simulink model "Comparacao_continuo_discreto"  (R2023b)
settings: Solver=FixedStepAuto  StartTime=0.0  StopTime=3  FixedStep=T  RelTol=1e-3
model workspace (MAT data in the model file):
  B = 0.0928996133407
  Cmn = 479.991198073
  I = 3000
  Ian = 260.13143483
  J = 0.56
  Kf = 1.91586963478
  La = 0.0014
  N = 3000
  Pele = 104052.573932
  Pmec = 95000
  Ra = 0.08
  T = 0.00175
  Te = 0.0175
  Tm = 6.02801217209
  Vn = 400
  Wn = 197.920296
libraries: simulink x1
settings Model: Creator=lpds  LastModifiedBy=USER

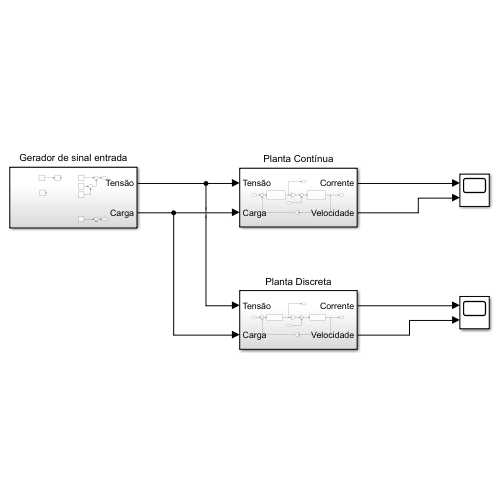
[thumbnail: Simulink's stored preview of the top-level diagram]
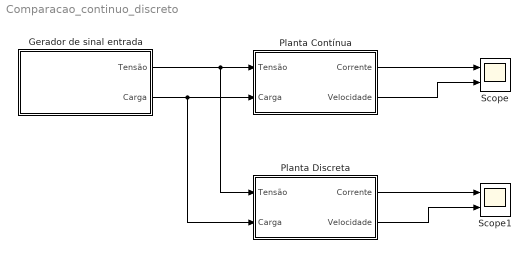
== system Comparacao_continuo_discreto ==
  Gerador de sinal entrada : Subsystem
  Planta Contínua : Subsystem
  Planta Discreta : Subsystem
  Scope : Scope  NumInputPorts=2
  Scope1 : Scope  NumInputPorts=2
  wires:
  Gerador de sinal entrada/1(Tensão) -> Planta Discreta/1(Tensão), Planta Contínua/1(Tensão)
  Gerador de sinal entrada/2(Carga) -> Planta Discreta/2(Carga), Planta Contínua/2(Carga)
  Planta Contínua/1(Corrente) -> Scope/1
  Planta Contínua/2(Velocidade) -> Scope/2
  Planta Discreta/1(Corrente) -> Scope1/1
  Planta Discreta/2(Velocidade) -> Scope1/2

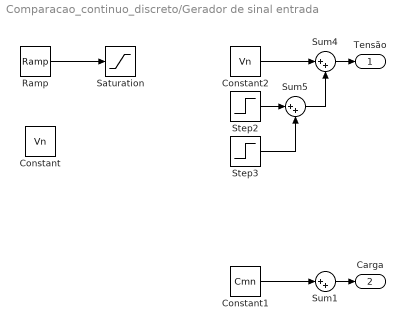
== system Comparacao_continuo_discreto/Gerador de sinal entrada ==
  Constant : Constant  Value=Vn
  Constant1 : Constant  Value=Cmn
  Constant2 : Constant  Value=Vn
  Ramp : simulink/Sources/Ramp  slope=Vn  start=0  InitialOutput=0
  Saturation : Saturate  UpperLimit=Vn  LowerLimit=0
  Step2 : Step  After=-50  SampleTime=0
  Step3 : Step  Time=2  After=100  SampleTime=0
  Sum1 : Sum  Inputs=|++
  Sum4 : Sum  Inputs=|++
  Sum5 : Sum  Inputs=|++
  Tensão : Outport
  Carga : Outport  Port=2
  wires:
  Constant1/1 -> Sum1/1
  Sum1/1 -> Carga/1
  Ramp/1 -> Saturation/1
  Constant2/1 -> Sum4/1
  Step3/1 -> Sum5/2
  Step2/1 -> Sum5/1
  Sum5/1 -> Sum4/2
  Sum4/1 -> Tensão/1

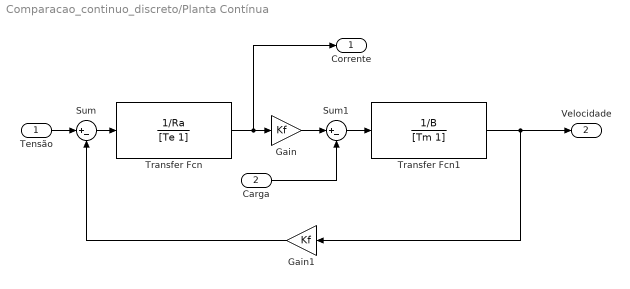
== system Comparacao_continuo_discreto/Planta Contínua ==
  Tensão : Inport
  Carga : Inport  Port=2
  Gain : Gain  Gain=Kf
  Gain1 : Gain  Gain=Kf
  Sum : Sum  Inputs=|+-
  Sum1 : Sum  Inputs=|+-
  Transfer Fcn : TransferFcn  Numerator=1/Ra  Denominator=[Te 1]
  Transfer Fcn1 : TransferFcn  Numerator=1/B  Denominator=[Tm 1]
  Corrente : Outport
  Velocidade : Outport  Port=2
  wires:
  Tensão/1 -> Sum/1
  Carga/1 -> Sum1/2
  Gain1/1 -> Sum/2
  Transfer Fcn1/1 -> Velocidade/1, Gain1/1
  Transfer Fcn/1 -> Corrente/1, Gain/1
  Gain/1 -> Sum1/1
  Sum/1 -> Transfer Fcn/1
  Sum1/1 -> Transfer Fcn1/1

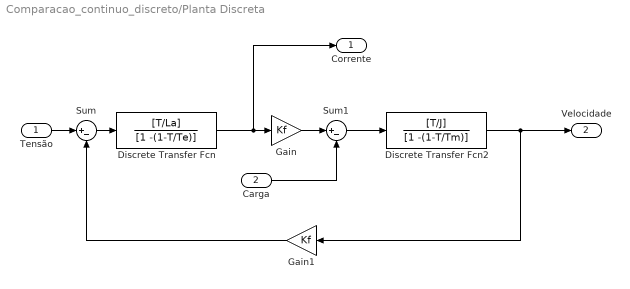
== system Comparacao_continuo_discreto/Planta Discreta ==
  Tensão : Inport
  Carga : Inport  Port=2
  Discrete Transfer Fcn : DiscreteTransferFcn  Numerator=[T/La]  Denominator=[1 -(1-T/Te)]
  Discrete Transfer Fcn2 : DiscreteTransferFcn  Numerator=[T/J]  Denominator=[1 -(1-T/Tm)]
  Gain : Gain  Gain=Kf
  Gain1 : Gain  Gain=Kf
  Sum : Sum  Inputs=|+-
  Sum1 : Sum  Inputs=|+-
  Corrente : Outport
  Velocidade : Outport  Port=2
  wires:
  Gain1/1 -> Sum/2
  Sum/1 -> Discrete Transfer Fcn/1
  Discrete Transfer Fcn2/1 -> Velocidade/1, Gain1/1
  Gain/1 -> Sum1/1
  Sum1/1 -> Discrete Transfer Fcn2/1
  Tensão/1 -> Sum/1
  Carga/1 -> Sum1/2
  Discrete Transfer Fcn/1 -> Corrente/1, Gain/1
